simulink model "Paper_plane_folding_withTime"  (R2024b)
settings: Solver=VariableStepAuto  StartTime=0.0  StopTime=100  RelTol=1e-3
undefined symbols (not defined in the file): m, n
settings Model: Creator=ruediger  LastModifiedBy=zainulhakimdalim
settings SolverCC: AlgebraicLoopSolver=TrustRegion
settings DataIOCC: SaveOutput=off  SaveTime=off
settings DebuggingCC: UnconnectedInputMsg=warning  UnconnectedOutputMsg=warning  UnconnectedLineMsg=warning  ArithmeticOperatorsInVariantConditions=warning
settings ModelReferenceCC: EnableRefExpFcnMdlSchedulingChecks=on
settings SFSimCC: SimUseLocalCustomCode=off  CustomCodeUndefinedFunction=UseInterfaceOnly
settings RTWCC: RTWUseLocalCustomCode=off  GPUComputeCapability=3.5
settings CodeAppCC: StateflowObjectComments=on

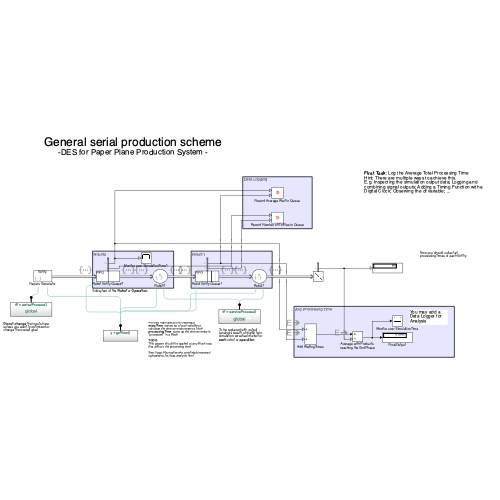
[thumbnail: Simulink's stored preview of the top-level diagram]
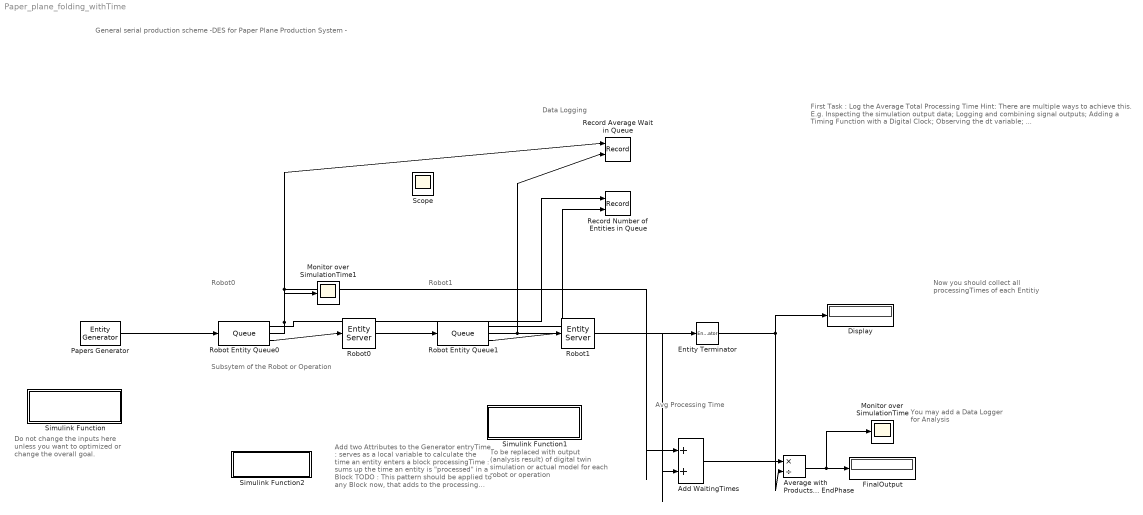
== system Paper_plane_folding_withTime ==
  note: Now you should collect all processingTimes of each Entitiy
  note: Avg Processing Time
  note: First Task : Log the Average Total Processing Time
      | Hint: There are multiple ways to achieve this.
      | E.g. Inspecting the simulation output data; Logging and combining signal outputs; Adding a Timing Function with a Digital Clock; Observing the dt variable; ...
  note: Subsytem of the Robot or Operation
  note: General serial production scheme
      | -DES for Paper Plane Production System -
  note: Data Logging
  note: Robot1
  note: Robot0
  note: Do not change the inputs here unless you want to optimized or change the overall goal.
  note: To be replaced with output (analysis result) of digital twin simulation or actual model for each robot or operation
  note: You may add a Data Logger for Analysis
  note: Add two Attributes to the Generator
      | entryTime : serves as a local variable to calculate the time an entity enters a block
      | processingTime : sums up the time an entity is "processed" in a Block
      |
      | TODO :
      | This pattern should be applied to any Block now, that adds to the processing time!
      |
      | See: https://de.mathworks.com/help/simevents/ug/statistics-for-data-analysis.html
  Add WaitingTimes : Sum
  Average with Products reaching the EndPhase : Product  Inputs=*/
  Display : Display
  Entity Terminator : EntityTerminator  InputPortMessageModes=m  NumberEntitiesArrived=on
      settings: OutputPortMap=o0
  FinalOutput : Display
  Monitor over SimulationTime : Scope
  Monitor over SimulationTime1 : Scope
  Papers Generator : EntityGenerator  OutputPortMessageModes=m  TimeSource=MATLAB action  IntergenerationTimeAction=dt = arrivalProcess();  GenerateAction=entity.entryTime0 = gettime();  AttributeName=entryTime0|processingTime0|entryTime1|processingTime1|executionTime0|executionTime1|entryTimerobot1|entryTimerobot0  AttributeInitialValue=0|0|0|0|0|0|0|0  EntityType=Structured  EntityTypeName=Entity
  Record Average Wait in Queue : Record  FileSettingsInternal="{\"entries\":[{\"content\":{\"excelSettings\":{\"content\":{},\"type\":\"Streamout.ExcelSettings\"}},\"type\":\"Streamout.FileSettingStorage\",\"uuid\":\"\"}],\"packageUris\":[\"http:\\/\\/schema.mathworks.com\\/mf0\\/streamout_blocks\\/R2020a\"],\"version\":\"1.0\"}"  SignalsInternal="{\"entries\":[{\"content\":{\"signals\":[{\"content\":{\"blockPath\":[],\"dimensions\":[1],\"domain\":\"\",\"lineColor\":\"#edb120\",\"lineWidth\":2,\"plots\":[ 1 ],\"port\":1,\"sid\":[\"\"],\"signalID\":1,\"signalName\":\"Robot Entity Queue0:2\"},\"type\":\"RecordBlkView.Signal\",\"uuid\":\"\"},{\"content\":{\"blockPath\":[],\"dimensions\":[1],\"domain\":\"\",\"lineColor\":\"#7e2f8e\",\"lineWidth\":2,\"plots\":[ 1 ],\"port\":2,\"sid\":[\"\"],\"signalID\":2,\"signalName\":\"Robot Entity Queue1:2\"},\"type\":\"RecordBlkView.Signal\",\"uuid\":\"\"}]},\"type\":\"RecordBlkView.InputSignals\",\"uuid\":\"\"}],\"packageUris\":[\"http:\\/\\/schema.mathworks.com\\/mf0\\/streamout_blocks\\/R2020a\"],\"version\":\"1.0\"}"  VisualizationBindings="{\"sparklinesplugin\":{\"info\":[{\"bindingParametersList\":[],\"subplotID\":1}]}}"
  Record Number of Entities in Queue : Record  FileSettingsInternal="{\"entries\":[{\"content\":{\"excelSettings\":{\"content\":{},\"type\":\"Streamout.ExcelSettings\"}},\"type\":\"Streamout.FileSettingStorage\",\"uuid\":\"\"}],\"packageUris\":[\"http:\\/\\/schema.mathworks.com\\/mf0\\/streamout_blocks\\/R2020a\"],\"version\":\"1.0\"}"  SignalsInternal="{\"entries\":[{\"content\":{\"signals\":[{\"content\":{\"blockPath\":[],\"dimensions\":[1],\"domain\":\"\",\"lineColor\":\"#a2142f\",\"lineWidth\":2,\"plots\":[ 1 ],\"port\":1,\"sid\":[\"\"],\"signalID\":1,\"signalName\":\"Robot Entity Queue0:1\"},\"type\":\"RecordBlkView.Signal\",\"uuid\":\"\"},{\"content\":{\"blockPath\":[],\"dimensions\":[1],\"domain\":\"\",\"lineColor\":\"#ff6929\",\"lineWidth\":2,\"plots\":[ 1 ],\"port\":2,\"sid\":[\"\"],\"signalID\":2,\"signalName\":\"Robot Entity Queue1:1\"},\"type\":\"RecordBlkView.Signal\",\"uuid\":\"\"}]},\"type\":\"RecordBlkView.InputSignals\",\"uuid\":\"\"}],\"packageUris\":[\"http:\\/\\/schema.mathworks.com\\/mf0\\/streamout_blocks\\/R2020a\"],\"version\":\"1.0\"}"  VisualizationBindings="{\"sparklinesplugin\":{\"info\":[{\"bindingParametersList\":[],\"subplotID\":1}]}}"
  Robot Entity Queue0 : Queue  InputPortMessageModes=m  OutputPortMessageModes=n,n,m  Capacity=inf  EntryAction=|  ExitAction=|  NumberEntitiesInBlock=on  AverageWait=on
      | % Time stamp for entity entry
      | entity.entryTime0 = gettime();
      | %persistent retain exitTime0 variable
      | persistent exitTime0 waitTimeArray0;
      | % Initialize the persistent array if empty
      | if isempty(waitTimeArray0)
      |     waitTimeArray0 = []; % Start with an empty array
      | end
      | 
      | % Time stamp for the entity exit 
      | exitTime0 = gettime();
      | % Duration between the entity entry and exit 
      | waitTime0 = exitTime0 - entity.entryTime0;
      | % Display the duration
      | %sprintf("This ist the waitTime0 %f ", waitTime0)
      | 
      | % Add it up
      | %entity.processingTime=entity-processingTime +waitTime
      | 
      | % Add the calculated waitTime0 to the array
      | waitTimeArray0 = [waitTimeArray0; waitTime0];
      | disp('This is the waitTimeArray0: ');
      | disp(waitTimeArray0);
      | 
      | % Save the waitTimeArray to the MATLAB workspace at the end of the simulation
      | assignin('base', 'waitTimeArray0', waitTimeArray0);
      settings: OutputPortMap=o1,o2,o5
  Robot Entity Queue1 : Queue  InputPortMessageModes=m  OutputPortMessageModes=n,n,m  Capacity=inf  EntryAction=|  ExitAction=|  NumberEntitiesInBlock=on  AverageWait=on
      | % Time stamp for entity entry
      | entity.entryTime1 = gettime();
      | %persistent retain exitTime0 variable
      | persistent exitTime1 waitTimeArray1;
      | % Initialize the persistent array if empty
      | if isempty(waitTimeArray1)
      |     waitTimeArray1 = []; % Start with an empty array
      | end
      | 
      | % Time stamp for the entity exit 
      | exitTime1 = gettime();
      | % Duration between the entity entry and exit 
      | waitTime1 = exitTime1 - entity.entryTime1;
      | % Display the duration
      | %sprintf("This ist the waitTime0 %f ", waitTime0)
      | 
      | % Add it up
      | %entity.processingTime=entity-processingTime +waitTime
      | 
      | % Add the calculated waitTime0 to the array
      | waitTimeArray1 = [waitTimeArray1; waitTime1];
      | disp('This is the waitTimeArray: ');
      | disp(waitTimeArray1);
      | 
      | % Save the waitTimeArray to the MATLAB workspace at the end of the simulation
      | assignin('base', 'waitTimeArray1', waitTimeArray1);
      settings: OutputPortMap=o1,o2,o5
  Robot0 : EntityServer  InputPortMessageModes=m  OutputPortMessageModes=m  Capacity=1  ServiceTimeSource=MATLAB action  ServiceTimeAction=dt = serviceProcess();  EntryAction=|  ServiceCompleteAction=|  ExitAction=|
      | % Time stamp for entity entry
      | entity.entryTimerobot0 = gettime();
      | % Time stamp for entity entry
      | entity.processingTime0 = gettime();
      | %persistent retain processTimerobot0 variable
      | persistent exitTimerobot0 processTimeArray0;
      | % Initialize the persistent array if empty
      | if isempty(processTimeArray0)
      |     processTimeArray0 = []; % Start with an empty array
      | end
      | 
      | % Time stamp for the entity exit 
      | exitTimerobot0 = gettime();
      | % Duration between the entity entry and exit 
      | processTimerobot0 = exitTimerobot0 - entity.entryTimerobot0;
      | % Display the duration
      | %sprintf("This ist the waitTime0 %f ", waitTime0)
      | 
      | % Add it up
      | %entity.processingTime=entity-processingTime +waitTime
      | 
      | % Add the calculated processTimerobot0 to the array
      | processTimeArray0 = [processTimeArray0; processTimerobot0];
      | disp('This is the processTimeArray0: ');
      | disp(processTimeArray0);
      | 
      | % Save the processTimeArray to the MATLAB workspace at the end of the simulation
      | assignin('base', 'processTimeArray0', processTimeArray0);
  Robot1 : EntityServer  InputPortMessageModes=m  OutputPortMessageModes=m  Capacity=1  ServiceTimeSource=MATLAB action  ServiceTimeAction=dt = serviceProcess();  EntryAction=|  ServiceCompleteAction=|  ExitAction=|
      | % Time stamp for entity entry
      | entity.entryTimerobot1 = gettime();
      | % Time stamp for entity entry
      | entity.processingTime1 = gettime();
      | %persistent retain processTimerobot0 variable
      | persistent exitTimerobot1 processTimeArray1;
      | % Initialize the persistent array if empty
      | if isempty(processTimeArray1)
      |     processTimeArray1 = []; % Start with an empty array
      | end
      | 
      | % Time stamp for the entity exit 
      | exitTimerobot1 = gettime();
      | % Duration between the entity entry and exit 
      | processTimerobot1 = exitTimerobot1 - entity.entryTimerobot1;
      | % Display the duration
      | %sprintf("This ist the waitTime0 %f ", waitTime0)
      | 
      | % Add it up
      | %entity.processingTime=entity-processingTime +waitTime
      | 
      | % Add the calculated processTimerobot0 to the array
      | processTimeArray1 = [processTimeArray1; processTimerobot1];
      | disp('This is the processTimeArray1: ');
      | disp(processTimeArray1);
      | 
      | % Save the processTimeArray to the MATLAB workspace at the end of the simulation
      | assignin('base', 'processTimeArray1', processTimeArray1);
  Simulink Function : Subsystem  TreatAsAtomicUnit=on
  Simulink Function1 : Subsystem  TreatAsAtomicUnit=on
  Simulink Function2 : Subsystem  TreatAsAtomicUnit=on
  Scope : Scope
  wires:
  Robot Entity Queue0/3 -> Robot0/1
  Papers Generator/1 -> Robot Entity Queue0/1
  Robot Entity Queue1/3 -> Robot1/1
  Robot0/1 -> Robot Entity Queue1/1
  Robot Entity Queue1/1 -> Record Number of Entities in Queue/2
  Robot Entity Queue0/1 -> Record Number of Entities in Queue/1
  Add WaitingTimes/1 -> Average with Products reaching the EndPhase/1
  Robot Entity Queue0/2 -> Monitor over SimulationTime1/1, Record Average Wait in Queue/1, Add WaitingTimes/1
  Average with Products reaching the EndPhase/1 -> Monitor over SimulationTime/1, FinalOutput/1
  Robot Entity Queue1/2 -> Add WaitingTimes/2, Record Average Wait in Queue/2
  Entity Terminator/1 -> Display/1, Average with Products reaching the EndPhase/2
  Robot1/1 -> Entity Terminator/1

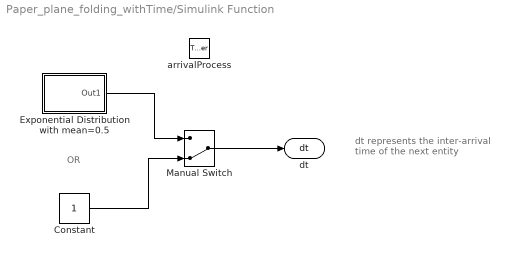
== system Paper_plane_folding_withTime/Simulink Function ==
  note: OR
  note: dt represents the inter-arrival time of the next entity
  arrivalProcess : TriggerPort  TriggerType=function-call  IsSimulinkFunction=on  FunctionName=arrivalProcess  VariantControl=Variant
  Constant : Constant
  Exponential Distribution with mean=0.5 : Subsystem
  Manual Switch : ManualSwitch  CurrentSetting=0
  dt : ArgOut  DisableCoverage=on  ArgumentName=dt
  wires:
  Manual Switch/1 -> dt/1
  Exponential Distribution with mean=0.5/1(Out1) -> Manual Switch/1
  Constant/1 -> Manual Switch/2

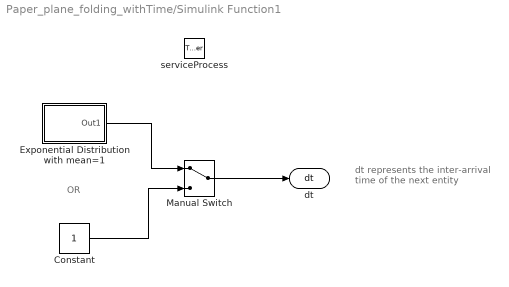
== system Paper_plane_folding_withTime/Simulink Function1 ==
  note: OR
  note: dt represents the inter-arrival time of the next entity
  serviceProcess : TriggerPort  TriggerType=function-call  IsSimulinkFunction=on  FunctionName=serviceProcess  VariantControl=Variant
  Constant : Constant
  Exponential Distribution with mean=1 : Subsystem
  Manual Switch : ManualSwitch
  dt : ArgOut  DisableCoverage=on  ArgumentName=dt
  wires:
  Manual Switch/1 -> dt/1
  Constant/1 -> Manual Switch/2
  Exponential Distribution with mean=1/1(Out1) -> Manual Switch/1

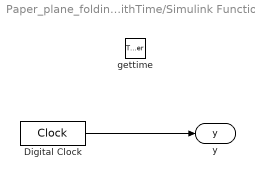
== system Paper_plane_folding_withTime/Simulink Function2 ==
  gettime : TriggerPort  TriggerType=function-call  IsSimulinkFunction=on  FunctionName=gettime  FunctionVisibility=scoped  VariantControl=(inherit)
  Digital Clock : DigitalClock  SampleTime=-1
  y : ArgOut  DisableCoverage=on  ArgumentName=y
  wires:
  Digital Clock/1 -> y/1

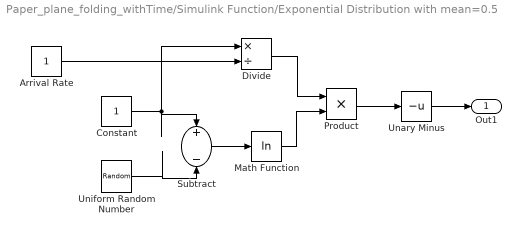
== system Paper_plane_folding_withTime/Simulink Function/Exponential Distribution with mean=0.5 ==
  Arrival Rate : Constant
  Constant : Constant
  Divide : Product  Inputs=*/
  Math Function : Math  Operator=log
  Product : Product
  Subtract : Sum  Inputs=+-
  Unary Minus : UnaryMinus
  Uniform Random Number : UniformRandomNumber  Minimum=0  Seed=12345
  Out1 : Outport
  wires:
  Unary Minus/1 -> Out1/1
  Arrival Rate/1 -> Divide/2
  Divide/1 -> Product/1
  Subtract/1 -> Math Function/1
  Math Function/1 -> Product/2
  Product/1 -> Unary Minus/1
  Uniform Random Number/1 -> Subtract/2
  Constant/1 -> Divide/1, Subtract/1

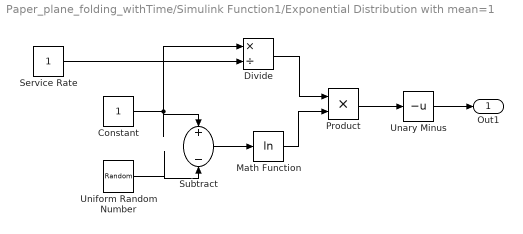
== system Paper_plane_folding_withTime/Simulink Function1/Exponential Distribution with mean=1 ==
  Constant : Constant
  Divide : Product  Inputs=*/
  Math Function : Math  Operator=log
  Product : Product
  Service Rate : Constant
  Subtract : Sum  Inputs=+-
  Unary Minus : UnaryMinus
  Uniform Random Number : UniformRandomNumber  Minimum=0  Seed=98765
  Out1 : Outport
  wires:
  Unary Minus/1 -> Out1/1
  Service Rate/1 -> Divide/2
  Divide/1 -> Product/1
  Subtract/1 -> Math Function/1
  Math Function/1 -> Product/2
  Product/1 -> Unary Minus/1
  Uniform Random Number/1 -> Subtract/2
  Constant/1 -> Divide/1, Subtract/1
